simulink model "pitchShift"  (R2022a)
settings: Solver=VariableStepAuto  StartTime=0.0  StopTime=18  RelTol=1e-3
PostLoadFcn:
  | postLoadCallback
InitFcn:
  | initCallback
StopFcn:
  | stopCallback
undefined symbols (not defined in the file or in its folder): modelParams
libraries: hdlsllib x4, embmathops x3, dspsrcs4 x2
CloseFcn:
  | closeCallback
settings Model: SimulationMode=accelerator  Creator=Ronnel  LastModifiedBy=Ronnel
settings DataIOCC: ReturnWorkspaceOutputs=off
settings OptimizationCC: BlockReduction=off  ConditionallyExecuteInputs=off  DefaultParameterBehavior=Inlined
settings DebuggingCC: AlgebraicLoopMsg=error
settings HardwareCC: ProdBitPerPointer=32  ProdBitPerSizeT=32  ProdBitPerPtrDiffT=32  ProdLargestAtomicFloat=None  ProdIntDivRoundTo=Undefined  ProdEndianess=Unspecified  ProdWordSize=32  ProdHWDeviceType=ASIC/FPGA->ASIC/FPGA  TargetBitPerPointer=64  TargetBitPerSizeT=64  TargetBitPerPtrDiffT=64  TargetLongLongMode=on  TargetIntDivRoundTo=Zero  TargetEndianess=LittleEndian  TargetWordSize=64  TargetHWDeviceType=Custom Processor->MATLAB Host Computer  ProdEqTarget=off

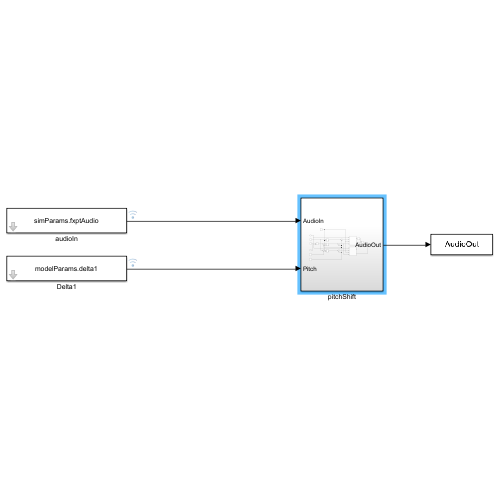
[thumbnail: Simulink's stored preview of the top-level diagram]
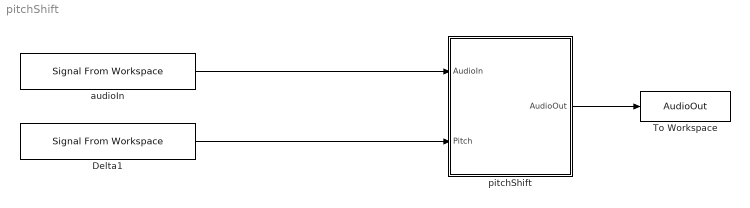
== system pitchShift ==
  Delta1 : dspsrcs4/Signal From Workspace  X=modelParams.delta1  Ts=modelParams.audio.samplePeriod  nsamps=1  OutputAfterFinalValue=Holding final value  ignoreOrWarnInputAndFrameLengths=off  OutputFrames=off
  To Workspace : ToWorkspace  VariableName=AudioOut  SampleTime=modelParams.audio.samplePeriod
      settings: Save2DSignal=2-D array (concatenate along first dimension)
  audioIn : dspsrcs4/Signal From Workspace  X=simParams.fxptAudio  Ts=modelParams.audio.samplePeriod  nsamps=1  OutputAfterFinalValue=Holding final value  ignoreOrWarnInputAndFrameLengths=off  OutputFrames=off
  pitchShift : Subsystem
  wires:
  audioIn/1 -> pitchShift/1(AudioIn)
  pitchShift/1(AudioOut) -> To Workspace/1
  Delta1/1 -> pitchShift/2(Pitch)

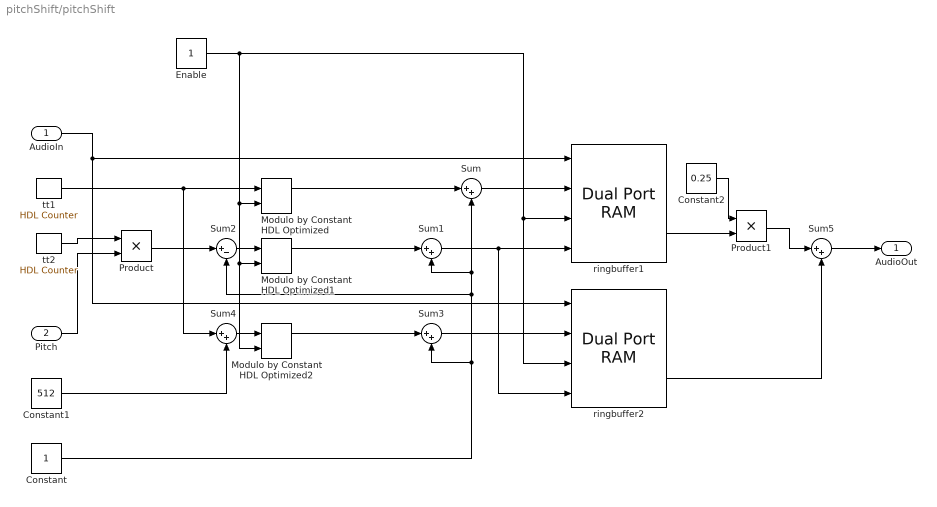
== system pitchShift/pitchShift ==
  AudioIn : Inport  SampleTime=modelParams.audio.samplePeriod
  Pitch : Inport  Port=2  SampleTime=modelParams.audio.samplePeriod
  Constant : Constant  OutDataTypeStr=uint32  SampleTime=modelParams.audio.samplePeriod
  Constant1 : Constant  Value=512  OutDataTypeStr=uint32  SampleTime=modelParams.audio.samplePeriod
  Constant2 : Constant  Value=0.25  OutDataTypeStr=fixdt(0,modelParams.audio.wordLength,modelParams.audio.fractionLength)  SampleTime=modelParams.audio.samplePeriod
  Enable : Constant  OutDataTypeStr=boolean  SampleTime=modelParams.audio.samplePeriod
  Modulo by Constant HDL Optimized : embmathops/Modulo by Constant HDL Optimized  Denominator=modelParams.buffer_size  SimulateUsing=Code generation
      settings: SourceProductBaseCode=SL
  Modulo by Constant HDL Optimized1 : embmathops/Modulo by Constant HDL Optimized  Denominator=modelParams.buffer_size  SimulateUsing=Code generation
      settings: SourceProductBaseCode=SL
  Modulo by Constant HDL Optimized2 : embmathops/Modulo by Constant HDL Optimized  Denominator=modelParams.buffer_size  SimulateUsing=Code generation
      settings: SourceProductBaseCode=SL
  Product : Product  SampleTime=modelParams.audio.samplePeriod
  Product1 : Product  OutDataTypeStr=fixdt(1,modelParams.audio.wordLength,modelParams.audio.fractionLength)  SaturateOnIntegerOverflow=on  SampleTime=modelParams.audio.samplePeriod
  Sum{,1,3..4} (4 alike) : Sum  Inputs=|++  OutDataTypeStr=fixdt(0,modelParams.dpramAddressSize,0)  SampleTime=modelParams.audio.samplePeriod
  Sum2 : Sum  Inputs=|+-  OutDataTypeStr=fixdt(0,modelParams.dpramAddressSize,0)  SampleTime=modelParams.audio.samplePeriod
  Sum5 : Sum  Inputs=|++  OutDataTypeStr=fixdt(1,modelParams.audio.wordLength,modelParams.audio.fractionLength)  SaturateOnIntegerOverflow=on  SampleTime=modelParams.audio.samplePeriod
  ringbuffer1 : hdlsllib/HDL RAMs/Dual Port RAM  ram_size=modelParams.dpramAddressSize
      settings: SourceProductBaseCode=SL
  ringbuffer2 : hdlsllib/HDL RAMs/Dual Port RAM  ram_size=modelParams.dpramAddressSize
      settings: SourceProductBaseCode=SL
  tt1 : hdlsllib/Sources/HDL Counter  CountType=Free running  CountInit=1  CountStep=1  CountMax=25  CountFromType=Initial value  CountFrom=1  CountResetPort=off  CountLoadPort=off  CountEnbPort=off  CountDirPort=off  CountHitOutputPort=off  CountDataType=Unsigned  CountWordLen=modelParams.dpramAddressSize  CountFracLen=0  CountSampTime=modelParams.audio.samplePeriod
  tt2 : hdlsllib/Sources/HDL Counter  CountType=Free running  CountInit=1  CountStep=1  CountMax=25  CountFromType=Initial value  CountFrom=1  CountResetPort=off  CountLoadPort=off  CountEnbPort=off  CountDirPort=off  CountHitOutputPort=off  CountDataType=Unsigned  CountWordLen=32  CountFracLen=0  CountSampTime=modelParams.audio.samplePeriod
  AudioOut : Outport  SampleTime=modelParams.audio.samplePeriod
  wires:
  Enable/1 -> Modulo by Constant HDL Optimized2/2, Modulo by Constant HDL Optimized1/2, Modulo by Constant HDL Optimized/2, ringbuffer1/3, ringbuffer2/3
  AudioIn/1 -> ringbuffer1/1, ringbuffer2/1
  tt1/1 -> Sum4/1, Modulo by Constant HDL Optimized/1
  Sum/1 -> ringbuffer1/2
  Constant/1 -> Sum3/2, Sum2/2, Sum1/2, Sum/2
  Modulo by Constant HDL Optimized/1 -> Sum/1
  Sum1/1 -> ringbuffer1/4, ringbuffer2/4
  Modulo by Constant HDL Optimized1/1 -> Sum1/1
  Sum2/1 -> Modulo by Constant HDL Optimized1/1
  tt2/1 -> Product/1
  Pitch/1 -> Product/2
  Product/1 -> Sum2/1
  Sum3/1 -> ringbuffer2/2
  Modulo by Constant HDL Optimized2/1 -> Sum3/1
  Sum4/1 -> Modulo by Constant HDL Optimized2/1
  Constant1/1 -> Sum4/2
  Constant2/1 -> Product1/1
  Product1/1 -> Sum5/1
  Sum5/1 -> AudioOut/1
  ringbuffer1/2 -> Product1/2
  ringbuffer2/2 -> Sum5/2
